simulink model "CommManager4SLX"  (R2023b)
settings: Solver=VariableStepAuto  StartTime=0.0  StopTime=10.0  RelTol=1e-3
libraries: instrumentlib x1, dspnetwork x1, slrealtimeiplib x1
settings Model: Creator=peterc  LastModifiedBy=peterc

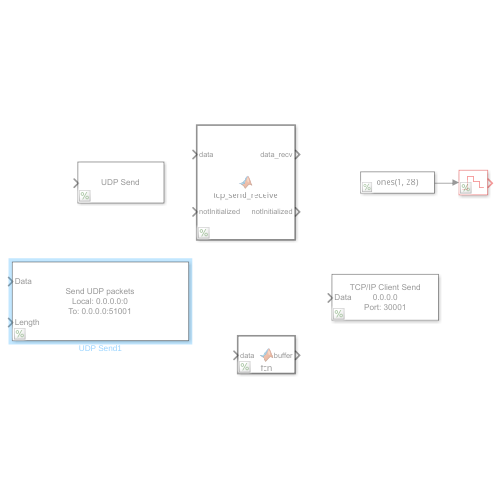
[thumbnail: Simulink's stored preview of the top-level diagram]
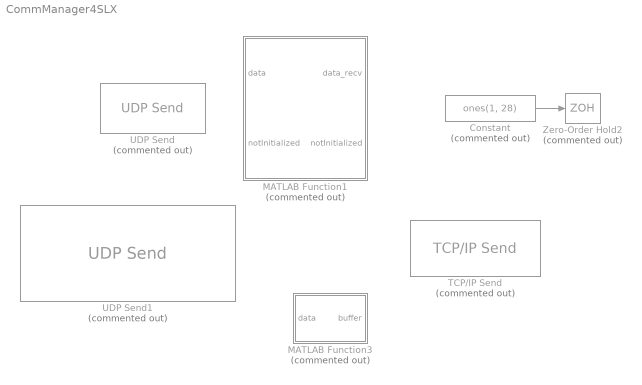
== system CommManager4SLX ==
  Constant : Constant  Commented=on  Value=ones(1, 28)  VectorParams1D=off  SampleTime=0.1
  MATLAB Function1 : MATLAB Function  Commented=on  TreatAsAtomicUnit=on
  MATLAB Function3 : MATLAB Function  Commented=on  TreatAsAtomicUnit=on
  TCP/IP Send : instrumentlib/TCP//IP Send  Commented=on  Host=0.0.0.0  Port=30001  ByteOrder=big-endian  EnableBlockingMode=off  Timeout=10  TransferDelay=on  SimulateUsing=Interpreted execution
  UDP Send : dspnetwork/UDP Send  Commented=on  remoteURL='0.0.0.0'  remotePort=51001  localURL='0.0.0.0'  localPortSource=Automatically determine  localPort=-1  sendBufferSize=224  sampletime=-1  blockPlatform=[]  separateLengthPort=0
      settings: LibrarySourceBlock=dspsnks4/UDP Send
  UDP Send1 : slrealtimeiplib/UDP Send  Commented=on  useHostTargetConn=off  toAddress='0.0.0.0'  toPort=51001  sampleTime=-1  enableMessage=off
  Zero-Order Hold2 : ZeroOrderHold  Commented=on  SampleTime=0.1
  wires:
  Constant/1 -> Zero-Order Hold2/1

== matlab function CommManager4SLX/MATLAB Function1 ==
  data: data input; data_recv output; notInitialized input; notInitialized output
function [data_recv, notInitialized] = tcp_send_receive(data, notInitialized)
    % MATLAB Function to send data via TCP and wait for a response
    % data: The data to send (from Simulink)
    % remoteHost: The remote server's IP address or hostname
    % remotePort: The remote server's port
    % localPort: The local port for the TCP client (optional)
    persistent tcpClient;

    num_bytes_recv = 12582912;
    remoteHost = 'localhost';
    remotePort = 30001;
    localPort = 30000;

    % Persistent TCP client for efficiency
    if notInitialized

        % Initialize TCP client if not already created
        if isempty(tcpClient)
            tcpClient = tcpclient(remoteHost, remotePort, 'LocalPort', localPort);
        end
        notInitialized = false;
    end

    % Send data
    write(tcpClient, data, 'uint8');
    
    % Read response
    data_recv = zeros(num_bytes_recv, 1);
    data_recv(:) = read(tcpClient, num_bytes_recv, 'uint8');

    % Cast to double

end

== matlab function CommManager4SLX/MATLAB Function3 ==
  data: data input; buffer output
function buffer = fcn(data)
buffer = zeros(1, 28*8, 'uint8');
buffer(:) = typecast(data, 'uint8');
end
